simulink model "point_1"  (R2022a)
settings: Solver=VariableStepAuto  StartTime=0.0  StopTime=T_sim  RelTol=1e-3
values from neighbouring files (symbols this model uses):
  A = [-1.2822  0      0.98     0 ... (first row only)    [main.m]
  B = [-0.3 ... (first row only)    [main.m]
  C = [0       1      0  0 ... (first row only)    [main.m]
  C_states = eye(length(A))    [main.m]
  D_states = zeros(length(B), 1)    [main.m]
  u_max = deg2rad(15)    [main.m]
  u_min = deg2rad(-15)    [main.m]
  x0 = [deg2rad(0) deg2rad(15) 0 -300]    [main.m]
  x_ref = [0 0 0 0]    [main.m]
undefined symbols (not defined in the file or in its folder): k_LQ1, k_LQ2, k_LQ3, k_LQ4
settings Model: Creator=PaoloA  LastModifiedBy=g_mor
settings DebuggingCC: UnconnectedInputMsg=warning  UnconnectedOutputMsg=warning  UnconnectedLineMsg=warning
settings RTWCC: DLArmComputeVersion=19.05

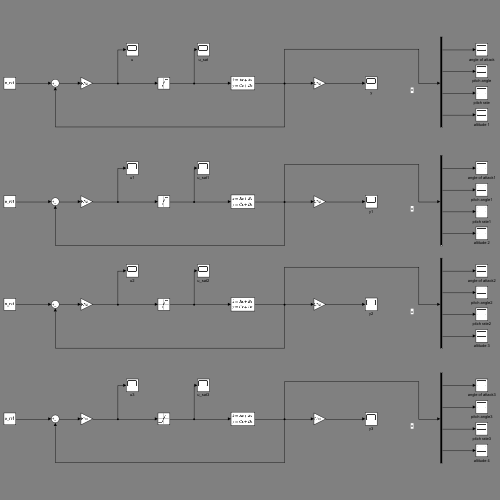
[thumbnail: Simulink's stored preview of the top-level diagram]
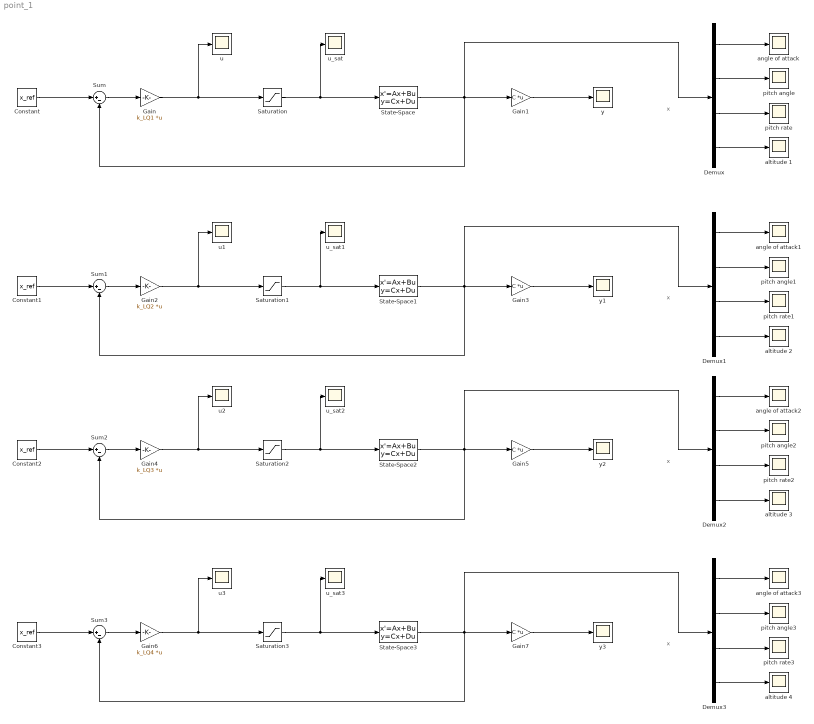
== system point_1 ==
  note: x
  note: x
  note: x
  note: x
  Constant{,1..3} (4 alike) : Constant  Value=x_ref
  Demux{,1..3} (4 alike) : Demux
  Gain : Gain  Gain=k_LQ1  Multiplication=Matrix(K*u)
  Gain{1,3,5,7} (4 alike) : Gain  Gain=C  Multiplication=Matrix(K*u)
  Gain2 : Gain  Gain=k_LQ2  Multiplication=Matrix(K*u)
  Gain4 : Gain  Gain=k_LQ3  Multiplication=Matrix(K*u)
  Gain6 : Gain  Gain=k_LQ4  Multiplication=Matrix(K*u)
  Saturation{,1..3} (4 alike) : Saturate  UpperLimit=u_max  LowerLimit=u_min
  State-Space{,1..3} (4 alike) : StateSpace  A=A  B=B  C=C_states  D=D_states  InitialCondition=x0
  Sum{,1..3} (4 alike) : Sum  Inputs=|+-
  altitude {1..4} (4 alike) : Scope
  angle of attack{,1..3} (4 alike) : Scope
  pitch angle{,1..3} (4 alike) : Scope
  pitch rate{,1..3} (4 alike) : Scope
  u{,1..3} (4 alike) : Scope
  u_sat{,1..3} (4 alike) : Scope
  y{,1..3} (4 alike) : Scope
  wires:
  Constant/1 -> Sum/1
  State-Space/1 -> Sum/2, Demux/1, Gain1/1
  Gain1/1 -> y/1
  Sum/1 -> Gain/1
  Gain/1 -> u/1, Saturation/1
  Saturation/1 -> u_sat/1, State-Space/1
  Demux/4 -> altitude 1/1
  Demux/3 -> pitch rate/1
  Demux/2 -> pitch angle/1
  Demux/1 -> angle of attack/1
  Demux1/4 -> altitude 2/1
  Demux1/3 -> pitch rate1/1
  Demux1/2 -> pitch angle1/1
  Demux1/1 -> angle of attack1/1
  Gain3/1 -> y1/1
  State-Space1/1 -> Sum1/2, Demux1/1, Gain3/1
  Sum1/1 -> Gain2/1
  Gain2/1 -> u1/1, Saturation1/1
  Constant1/1 -> Sum1/1
  Saturation1/1 -> u_sat1/1, State-Space1/1
  Gain4/1 -> u2/1, Saturation2/1
  Constant2/1 -> Sum2/1
  Sum2/1 -> Gain4/1
  Saturation2/1 -> u_sat2/1, State-Space2/1
  State-Space2/1 -> Sum2/2, Demux2/1, Gain5/1
  Demux2/2 -> pitch angle2/1
  Demux2/1 -> angle of attack2/1
  Demux2/3 -> pitch rate2/1
  Demux2/4 -> altitude 3/1
  Gain5/1 -> y2/1
  Gain6/1 -> u3/1, Saturation3/1
  Constant3/1 -> Sum3/1
  Sum3/1 -> Gain6/1
  Saturation3/1 -> u_sat3/1, State-Space3/1
  State-Space3/1 -> Sum3/2, Demux3/1, Gain7/1
  Demux3/2 -> pitch angle3/1
  Demux3/1 -> angle of attack3/1
  Demux3/3 -> pitch rate3/1
  Demux3/4 -> altitude 4/1
  Gain7/1 -> y3/1
